simulink model "SS_Serial"  (R2019b)
settings: Solver=VariableStepAuto  StartTime=0.0  StopTime=60.0  FixedStep=0.00000001  RelTol=1e-3
undefined symbols (not defined in the file): __PRM__SERIALIZED__DATA__, SubsystemReferenceBlock
settings Model: Creator=toons  LastModifiedBy=toons
settings DataIOCC: ExternalInput=[input1, input2]  ReturnWorkspaceOutputs=off
settings DebuggingCC: ArithmeticOperatorsInVariantConditions=warning
settings SFSimCC: CustomCodeUndefinedFunction=UseInterfaceOnly

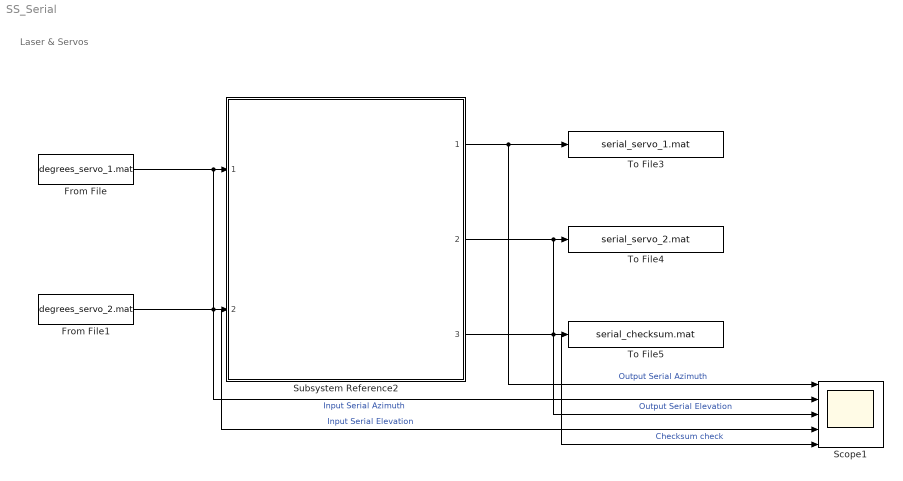
== system SS_Serial ==
  note: Laser & Servos
  From File : FromFile  FileName=degrees_servo_1.mat  SampleTime=0.0001  ExtrapolationBeforeFirstDataPoint=Hold first value  InterpolationWithinTimeRange=Zero order hold  ExtrapolationAfterLastDataPoint=Hold last value
  From File1 : FromFile  FileName=degrees_servo_2.mat  SampleTime=0.0001  ExtrapolationBeforeFirstDataPoint=Hold first value  InterpolationWithinTimeRange=Zero order hold  ExtrapolationAfterLastDataPoint=Hold last value
  Scope1 : Scope  NumInputPorts=5
  Subsystem Reference2 : Subsystem  BlockKeywords=__PRM__SERIALIZED__DATA__:SubsystemReferenceBlock  ReferencedSubsystem=SerialCommunication
  To File3 : ToFile  Filename=serial_servo_1.mat  SaveFormat=Timeseries
  To File4 : ToFile  Filename=serial_servo_2.mat  SaveFormat=Timeseries
  To File5 : ToFile  Filename=serial_checksum.mat  SaveFormat=Timeseries
  wires:
  From File/1 -> Scope1/2, Subsystem Reference2/1  "Input Serial Azimuth"
  From File1/1 -> Scope1/4, Subsystem Reference2/2  "Input Serial Elevation"
  Subsystem Reference2/1 -> Scope1/1, To File3/1  "Output Serial Azimuth"
  Subsystem Reference2/2 -> Scope1/3, To File4/1  "Output Serial Elevation"
  Subsystem Reference2/3 -> Scope1/5, To File5/1  "Checksum check"
